simulink subsystem "EDT_Environmental_Models"  (R2024a)
settings: Solver=VariableStepAuto  StartTime=0.0  StopTime=10.0  RelTol=1e-3
undefined symbols (not defined in the file): tether
libraries: matrix_library x2, aerolibtransform2 x1
settings Model: Creator=dani  LastModifiedBy=dani

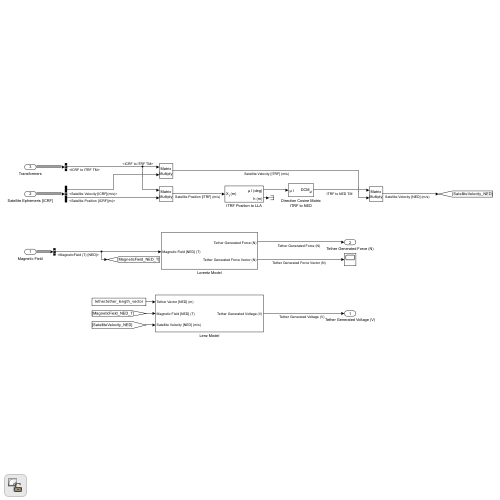
[thumbnail: Simulink's stored preview of the top-level diagram]
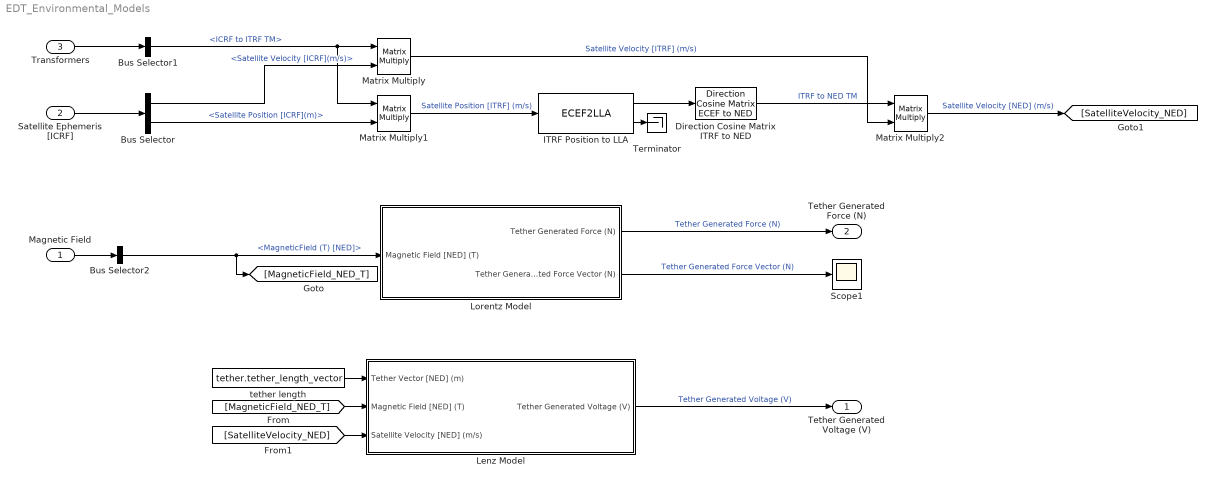
== system EDT_Environmental_Models ==
  Magnetic Field : Inport
  Satellite Ephemeris [ICRF] : Inport  Port=2
  Transformers : Inport  Port=3
  Bus Selector : BusSelector  OutputSignals=Satellite Ephemeris [ICRF].Satellite Velocity [ICRF](m/s),Satellite Ephemeris [ICRF].Satellite Position [ICRF](m)
  Bus Selector1 : BusSelector  OutputSignals=Transfer Matrices.ICRF to ITRF TM
  Bus Selector2 : BusSelector  OutputSignals=MagneticField (T) [NED]
  Direction Cosine Matrix ITRF to NED : aerolibtransform2/Direction Cosine Matrix ECEF to NED
  ITRF Position to LLA : ECEF2LLA
  Lenz Model : Subsystem
  Lorentz Model : Subsystem
  Matrix Multiply : Product  Multiplication=Matrix(*)
  Matrix Multiply1 : Product  Multiplication=Matrix(*)
  Matrix Multiply2 : Product  Multiplication=Matrix(*)
  Scope1 : Scope
  Terminator : Terminator
  tether length : Constant  Value=tether.tether_length_vector
  Tether Generated Voltage (V) : Outport
  Tether Generated Force (N) : Outport  Port=2
  wires:
  Transformers/1 -> Bus Selector1/1
  Satellite Ephemeris [ICRF]/1 -> Bus Selector/1
  Bus Selector1/1 -> Matrix Multiply/1, Matrix Multiply1/1  "<ICRF to ITRF TM>"
  ITRF Position to LLA/1 -> Direction Cosine Matrix ITRF to NED/1
  Bus Selector/1 -> Matrix Multiply/2  "<Satellite Velocity [ICRF](m/s)>"
  Matrix Multiply/1 -> Matrix Multiply2/2  "Satellite Velocity [ITRF] (m/s)"
  ITRF Position to LLA/2 -> Terminator/1
  Magnetic Field/1 -> Bus Selector2/1
  Bus Selector2/1 -> Lorentz Model/1(Magnetic Field [NED] (T)), [MagneticField_NED_T]  "<MagneticField (T) [NED]>"
  Lorentz Model/1(Tether Generated Force (N)) -> Tether Generated Force (N)/1  "Tether Generated Force (N)"
  Direction Cosine Matrix ITRF to NED/1 -> Matrix Multiply2/1  "ITRF to NED TM"
  Lenz Model/1(Tether Generated Voltage (V)) -> Tether Generated Voltage (V)/1  "Tether Generated Voltage (V)"
  [MagneticField_NED_T] -> Lenz Model/2(Magnetic Field [NED] (T))
  tether length/1 -> Lenz Model/1(Tether Vector [NED] (m))
  Lorentz Model/2(Tether Generated Force Vector (N)) -> Scope1/1  "Tether Generated Force Vector (N)"
  Bus Selector/2 -> Matrix Multiply1/2  "<Satellite Position [ICRF](m)>"
  Matrix Multiply1/1 -> ITRF Position to LLA/1  "Satellite Position [ITRF] (m/s)"
  Matrix Multiply2/1 -> [SatelliteVelocity_NED]  "Satellite Velocity [NED] (m/s)"
  [SatelliteVelocity_NED] -> Lenz Model/3(Satellite Velocity [NED] (m/s))

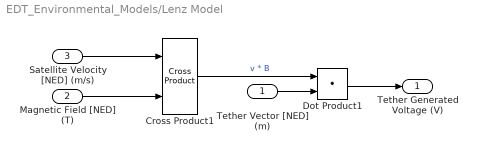
== system EDT_Environmental_Models/Lenz Model ==
  Tether Vector [NED] (m) : Inport
  Magnetic Field [NED] (T) : Inport  Port=2
  Satellite Velocity [NED] (m/s) : Inport  Port=3
  Cross Product1 : matrix_library/Cross Product
  Dot Product1 : DotProduct  OutDataTypeStr=Inherit: Inherit via internal rule
  Tether Generated Voltage (V) : Outport
  wires:
  Dot Product1/1 -> Tether Generated Voltage (V)/1
  Tether Vector [NED] (m)/1 -> Dot Product1/2
  Magnetic Field [NED] (T)/1 -> Cross Product1/2
  Satellite Velocity [NED] (m/s)/1 -> Cross Product1/1
  Cross Product1/1 -> Dot Product1/1  "v * B"

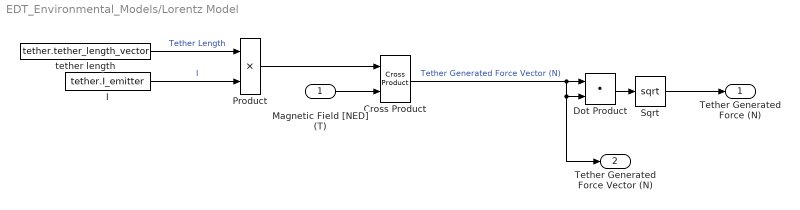
== system EDT_Environmental_Models/Lorentz Model ==
  Magnetic Field [NED] (T) : Inport
  Cross Product : matrix_library/Cross Product
  Dot Product : DotProduct  OutDataTypeStr=Inherit: Inherit via internal rule
  "I " : Constant  Value=tether.I_emitter
  Product : Product
  Sqrt : Sqrt
  tether length : Constant  Value=tether.tether_length_vector
  Tether Generated Force (N) : Outport
  Tether Generated Force Vector (N) : Outport  Port=2
  wires:
  Cross Product/1 -> Dot Product/1, Tether Generated Force Vector (N)/1, Dot Product/2  "Tether Generated Force Vector (N)"
  "I "/1 -> Product/2  "I"
  Dot Product/1 -> Sqrt/1
  Sqrt/1 -> Tether Generated Force (N)/1
  Magnetic Field [NED] (T)/1 -> Cross Product/2
  tether length/1 -> Product/1  "Tether Length"
  Product/1 -> Cross Product/1
